simulink model "FOC_6EKF_V2"  (R2024b)
settings: Solver=ode4  StartTime=0.0  StopTime=20  FixedStep=1e-6  RelTol=1e-3
libraries: spsMosfetLib x6, simulink x4, mcbcontrolslib x4, slpidlib x3, eeGeneralControl x3, spsSeriesRLCBranchLib x2, spsPermanentMagnetSynchronousMachineLib x1, sps_lib x1, spsDCVoltageSourceLib x1
settings Model: SimulationMode=accelerator  Creator=谭恩泽  LastModifiedBy=谭恩泽

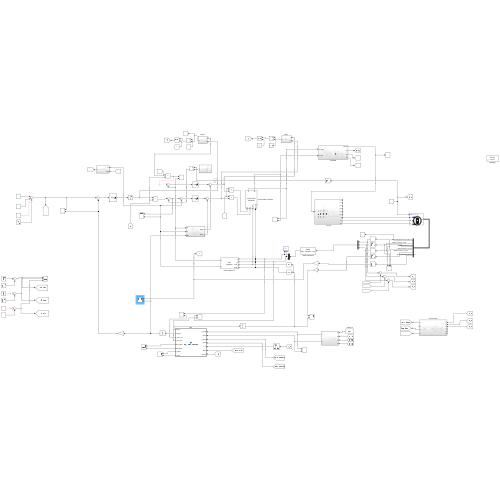
[thumbnail: Simulink's stored preview of the top-level diagram]
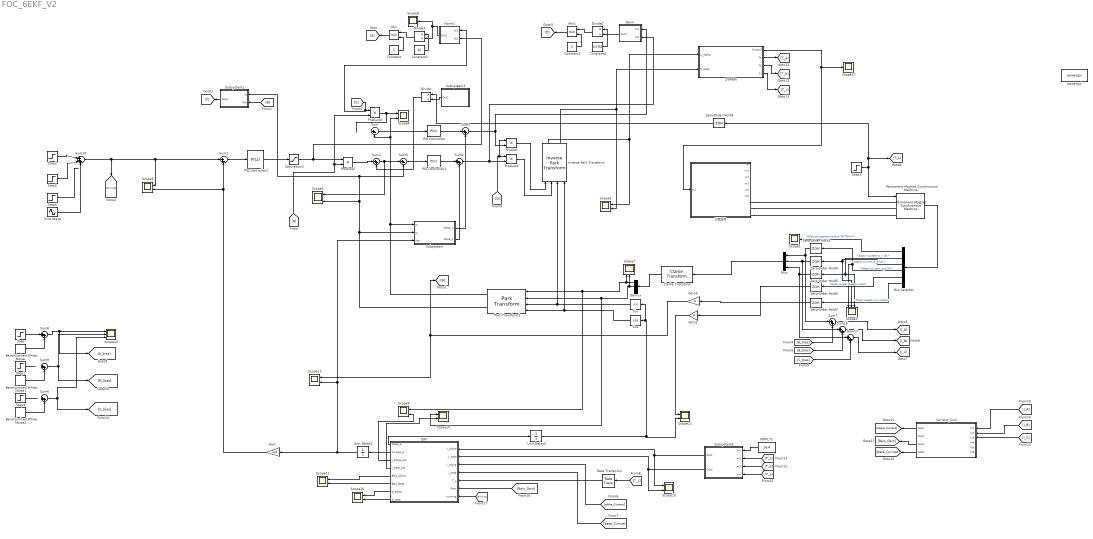
== system FOC_6EKF_V2 ==
  Band-Limited White Noise : simulink/Sources/Band-Limited White Noise  Cov=[1e-8]  Ts=1e-4  seed=[23341]
  Band-Limited White Noise1 : simulink/Sources/Band-Limited White Noise  Cov=[1e-8]  Ts=1e-4  seed=[23341]
  Band-Limited White Noise2 : simulink/Sources/Band-Limited White Noise  Cov=[1e-8]  Ts=1e-4  seed=[23341]
  Bus Selector : BusSelector  OutputSignals=Electromagnetic torque Te (N*m),Stator current is_c (A),Stator current is_b (A),Stator current is_a (A),Rotor angle thetam (rad),Rotor speed wm (rad/s)
  Clarke Transform : mcbcontrolslib/Clarke Transform  VariantControl=Variant2  PhaseInput=Three inputs  EnPowerInv=off
      settings: LibrarySourceBlock=mcblib/Controls/Math Transforms/Clarke Transform
  Constant : Constant  SampleTime=1e-4
  Constant1 : Constant  Value=20  SampleTime=1e-4
  Constant2 : Constant  SampleTime=1e-4
  Constant4 : Constant  Value=13.84  SampleTime=1e-4
  Cos : Trigonometry  Operator=cos
  Current_Sum : Subsystem
  Demux : Demux  Outputs=3
  Divide : Product  Inputs=*/  SampleTime=1e-4
  Divide1 : Product  Inputs=*/  SampleTime=1e-4
  Divide2 : Product  Inputs=*/  SampleTime=1e-4
  EKF : MATLAB Function  TreatAsAtomicUnit=on  SystemSampleTime=1e-4
  From : From
  Gain : Gain  Gain=1/4
  Gain2 : Gain  Gain=4
  Gain3 : Gain  Gain=4
  Goto : Goto
  Inverse Park Transform : mcbcontrolslib/Inverse Park Transform  PhaseInput=Two inputs  AxisAlignment=D-axis  ThetaInput=Sine and Cosine electrical position  AngleInput=Radians  N_points=1024
      settings: LibrarySourceBlock=mcblib/Controls/Math Transforms/Inverse Park Transform
  Min : MinMax  Inputs=2  SampleTime=1e-4
  Min1 : MinMax  Inputs=2  SampleTime=1e-4
  Mux : Mux  Inputs=3
  Norm : Subsystem
  Norm1 : Subsystem
  PID Controller : slpidlib/PID Controller  Controller=PI  Form=Parallel  TimeDomain=Discrete-time  UseExternalTs=off  SampleTime=1e-4  IntegratorMethod=Forward Euler  FilterMethod=Forward Euler  ControllerParametersSource=internal  P=3  I=0.5  UseKiTs=on  D=0  UseExternalDerivativeSource=off  N=100  UseFilter=on  TunerSelectOption=Transfer Function Based (PID Tuner App)  InitialConditionSource=internal  InitialConditionForIntegrator=0  InitialConditionForFilter=0  DifferentiatorICPrevScaledInput=0  ExternalReset=none  TrackingMode=off  Kt=1  LimitOutput=on  SatLimitsSource=internal  UpperSaturationLimit=15  LowerSaturationLimit=-15  LinearizeAsGain=on  AntiWindupMode=clamping  Kb=1  LimitIntegrator=off  UpperIntegratorSaturationLimit=inf  LowerIntegratorSaturationLimit=-inf  POutMin=[]  POutMax=[]  IOutMin=[]  IOutMax=[]  DOutMin=[]  DOutMax=[]  NOutMin=[]  NOutMax=[]  SumOutMin=[]  SumOutMax=[]  SaturationOutMin=[]  SaturationOutMax=[]  PParamMin=[]  PParamMax=[]  IParamMin=[]  IParamMax=[]  DParamMin=[]  DParamMax=[]  NParamMin=[]  NParamMax=[]  KbParamMin=[]  KbParamMax=[]  KtParamMin=[]  KtParamMax=[]  KbOutMin=[]  KbOutMax=[]  KtOutMin=[]  KtOutMax=[]  IntegratorOutMin=[]  IntegratorOutMax=[]  FilterOutMin=[]  FilterOutMax=[]  SumI1OutMin=[]  SumI1OutMax=[]  SumI2OutMin=[]  SumI2OutMax=[]  SumI3OutMin=[]  SumI3OutMax=[]  SumI4OutMin=[]  SumI4OutMax=[]  SumDOutMin=[]  SumDOutMax=[]  DifferentiatorOutMin=[]  DifferentiatorOutMax=[]  FilterDiffOutCoefMin=[]  FilterDiffOutCoefMax=[]  ReciprocalOutMin=[]  ReciprocalOutMax=[]  SumDenOutMin=[]  SumDenOutMax=[]  SumNumOutMin=[]  SumNumOutMax=[]  DivideOutMin=[]  DivideOutMax=[]  UdiffTsProdOutMin=[]  UdiffTsProdOutMax=[]  NTsProdOutMin=[]  NTsProdOutMax=[]  UintegralTsProdOutMin=[]  UintegralTsProdOutMax=[]  UngainTsProdOutMin=[]  UngainTsProdOutMax=[]  ClampingZeroOutDataTypeStr=Inherit: Inherit via back propagation  ClampingZeroOutMin=[]  ClampingZeroOutMax=[]  FilterDenConstantOutDataTypeStr=Inherit: Inherit via back propagation  FilterDenConstantOutMin=[]  FilterDenConstantOutMax=[]  PCopyOutDataTypeStr=Inherit: Inherit via back propagation  PCopyOutMin=[]  PCopyOutMax=[]  NCopyOutDataTypeStr=Inherit: Inherit via back propagation  NCopyOutMin=[]  NCopyOutMax=[]  IntegratorContinuousStateAttributes=''  IntegratorStateMustResolveToSignalObject=off  IntegratorRTWStateStorageClass=Auto  FilterContinuousStateAttributes=''  FilterStateMustResolveToSignalObject=off  FilterRTWStateStorageClass=Auto  ParallelPVariant=InternalParameters  IdealPVariant=Disabled  IVariant=InternalParameters  DVariant=Disabled  IntegratorVariant=Discrete  SatVariant=Enabled  AWVariant=DiscClampingParallel  PCopyVariant=Disabled  TRVariant=Disabled  FdbkBlocksVariant=Forward  IdealPFdbkVariant=Disabled  SatFdbkVariant=Disabled  DerivativeFilterVariant=Disabled  NVariant=Disabled  NCopyVariant=Disabled_SignalSpec  FilterICVariant=Disabled  IntegratorICVariant=InternalICs  ExternalResetVariant=Disabled  TRSumVariant=Passthrough  SumFdbkVariant=Disabled  SumVariant=Sum_PI  TsampFilterVariant=InternalTs  TsampNgainVariant=Passthrough  TsampIntegralVariant=Disabled_SignalSpec  ExternalSaturationOutDataTypeStr=Inherit: Same as second input  DerivativeSourceVariant=Disabled  PreIntVariant=InternalPreInt
  PID Controller1 : slpidlib/PID Controller  Controller=PI  Form=Parallel  TimeDomain=Discrete-time  UseExternalTs=off  SampleTime=1e-4  IntegratorMethod=Forward Euler  FilterMethod=Forward Euler  ControllerParametersSource=internal  P=3  I=0.5  UseKiTs=on  D=0  UseExternalDerivativeSource=off  N=100  UseFilter=on  TunerSelectOption=Transfer Function Based (PID Tuner App)  InitialConditionSource=internal  InitialConditionForIntegrator=0  InitialConditionForFilter=0  DifferentiatorICPrevScaledInput=0  ExternalReset=none  TrackingMode=off  Kt=1  LimitOutput=on  SatLimitsSource=internal  UpperSaturationLimit=15  LowerSaturationLimit=-15  LinearizeAsGain=on  AntiWindupMode=clamping  Kb=1  LimitIntegrator=off  UpperIntegratorSaturationLimit=inf  LowerIntegratorSaturationLimit=-inf  POutMin=[]  POutMax=[]  IOutMin=[]  IOutMax=[]  DOutMin=[]  DOutMax=[]  NOutMin=[]  NOutMax=[]  SumOutMin=[]  SumOutMax=[]  SaturationOutMin=[]  SaturationOutMax=[]  PParamMin=[]  PParamMax=[]  IParamMin=[]  IParamMax=[]  DParamMin=[]  DParamMax=[]  NParamMin=[]  NParamMax=[]  KbParamMin=[]  KbParamMax=[]  KtParamMin=[]  KtParamMax=[]  KbOutMin=[]  KbOutMax=[]  KtOutMin=[]  KtOutMax=[]  IntegratorOutMin=[]  IntegratorOutMax=[]  FilterOutMin=[]  FilterOutMax=[]  SumI1OutMin=[]  SumI1OutMax=[]  SumI2OutMin=[]  SumI2OutMax=[]  SumI3OutMin=[]  SumI3OutMax=[]  SumI4OutMin=[]  SumI4OutMax=[]  SumDOutMin=[]  SumDOutMax=[]  DifferentiatorOutMin=[]  DifferentiatorOutMax=[]  FilterDiffOutCoefMin=[]  FilterDiffOutCoefMax=[]  ReciprocalOutMin=[]  ReciprocalOutMax=[]  SumDenOutMin=[]  SumDenOutMax=[]  SumNumOutMin=[]  SumNumOutMax=[]  DivideOutMin=[]  DivideOutMax=[]  UdiffTsProdOutMin=[]  UdiffTsProdOutMax=[]  NTsProdOutMin=[]  NTsProdOutMax=[]  UintegralTsProdOutMin=[]  UintegralTsProdOutMax=[]  UngainTsProdOutMin=[]  UngainTsProdOutMax=[]  ClampingZeroOutDataTypeStr=Inherit: Inherit via back propagation  ClampingZeroOutMin=[]  ClampingZeroOutMax=[]  FilterDenConstantOutDataTypeStr=Inherit: Inherit via back propagation  FilterDenConstantOutMin=[]  FilterDenConstantOutMax=[]  PCopyOutDataTypeStr=Inherit: Inherit via back propagation  PCopyOutMin=[]  PCopyOutMax=[]  NCopyOutDataTypeStr=Inherit: Inherit via back propagation  NCopyOutMin=[]  NCopyOutMax=[]  IntegratorContinuousStateAttributes=''  IntegratorStateMustResolveToSignalObject=off  IntegratorRTWStateStorageClass=Auto  FilterContinuousStateAttributes=''  FilterStateMustResolveToSignalObject=off  FilterRTWStateStorageClass=Auto  ParallelPVariant=InternalParameters  IdealPVariant=Disabled  IVariant=InternalParameters  DVariant=Disabled  IntegratorVariant=Discrete  SatVariant=Enabled  AWVariant=DiscClampingParallel  PCopyVariant=Disabled  TRVariant=Disabled  FdbkBlocksVariant=Forward  IdealPFdbkVariant=Disabled  SatFdbkVariant=Disabled  DerivativeFilterVariant=Disabled  NVariant=Disabled  NCopyVariant=Disabled_SignalSpec  FilterICVariant=Disabled  IntegratorICVariant=InternalICs  ExternalResetVariant=Disabled  TRSumVariant=Passthrough  SumFdbkVariant=Disabled  SumVariant=Sum_PI  TsampFilterVariant=InternalTs  TsampNgainVariant=Passthrough  TsampIntegralVariant=Disabled_SignalSpec  ExternalSaturationOutDataTypeStr=Inherit: Same as second input  DerivativeSourceVariant=Disabled  PreIntVariant=InternalPreInt
  PID Controller2 : slpidlib/PID Controller  Controller=PI  Form=Parallel  TimeDomain=Discrete-time  UseExternalTs=off  SampleTime=1e-4  IntegratorMethod=Forward Euler  FilterMethod=Forward Euler  ControllerParametersSource=internal  P=1.2  I=0.002  UseKiTs=on  D=0  UseExternalDerivativeSource=off  N=100  UseFilter=off  TunerSelectOption=Transfer Function Based (PID Tuner App)  InitialConditionSource=internal  InitialConditionForIntegrator=0  InitialConditionForFilter=0  DifferentiatorICPrevScaledInput=0  ExternalReset=none  TrackingMode=off  Kt=1  LimitOutput=on  SatLimitsSource=internal  UpperSaturationLimit=20  LowerSaturationLimit=-20  LinearizeAsGain=on  AntiWindupMode=clamping  Kb=1  LimitIntegrator=off  UpperIntegratorSaturationLimit=inf  LowerIntegratorSaturationLimit=-inf  POutMin=[]  POutMax=[]  IOutMin=[]  IOutMax=[]  DOutMin=[]  DOutMax=[]  NOutMin=[]  NOutMax=[]  SumOutMin=[]  SumOutMax=[]  SaturationOutMin=[]  SaturationOutMax=[]  PParamMin=[]  PParamMax=[]  IParamMin=[]  IParamMax=[]  DParamMin=[]  DParamMax=[]  NParamMin=[]  NParamMax=[]  KbParamMin=[]  KbParamMax=[]  KtParamMin=[]  KtParamMax=[]  KbOutMin=[]  KbOutMax=[]  KtOutMin=[]  KtOutMax=[]  IntegratorOutMin=[]  IntegratorOutMax=[]  FilterOutMin=[]  FilterOutMax=[]  SumI1OutMin=[]  SumI1OutMax=[]  SumI2OutMin=[]  SumI2OutMax=[]  SumI3OutMin=[]  SumI3OutMax=[]  SumI4OutMin=[]  SumI4OutMax=[]  SumDOutMin=[]  SumDOutMax=[]  DifferentiatorOutMin=[]  DifferentiatorOutMax=[]  FilterDiffOutCoefMin=[]  FilterDiffOutCoefMax=[]  ReciprocalOutMin=[]  ReciprocalOutMax=[]  SumDenOutMin=[]  SumDenOutMax=[]  SumNumOutMin=[]  SumNumOutMax=[]  DivideOutMin=[]  DivideOutMax=[]  UdiffTsProdOutMin=[]  UdiffTsProdOutMax=[]  NTsProdOutMin=[]  NTsProdOutMax=[]  UintegralTsProdOutMin=[]  UintegralTsProdOutMax=[]  UngainTsProdOutMin=[]  UngainTsProdOutMax=[]  ClampingZeroOutDataTypeStr=Inherit: Inherit via back propagation  ClampingZeroOutMin=[]  ClampingZeroOutMax=[]  FilterDenConstantOutDataTypeStr=Inherit: Inherit via back propagation  FilterDenConstantOutMin=[]  FilterDenConstantOutMax=[]  PCopyOutDataTypeStr=Inherit: Inherit via back propagation  PCopyOutMin=[]  PCopyOutMax=[]  NCopyOutDataTypeStr=Inherit: Inherit via back propagation  NCopyOutMin=[]  NCopyOutMax=[]  IntegratorContinuousStateAttributes=''  IntegratorStateMustResolveToSignalObject=off  IntegratorRTWStateStorageClass=Auto  FilterContinuousStateAttributes=''  FilterStateMustResolveToSignalObject=off  FilterRTWStateStorageClass=Auto  ParallelPVariant=InternalParameters  IdealPVariant=Disabled  IVariant=InternalParameters  DVariant=Disabled  IntegratorVariant=Discrete  SatVariant=Enabled  AWVariant=DiscClampingParallel  PCopyVariant=Disabled  TRVariant=Disabled  FdbkBlocksVariant=Forward  IdealPFdbkVariant=Disabled  SatFdbkVariant=Disabled  DerivativeFilterVariant=Disabled  NVariant=Disabled  NCopyVariant=Disabled_SignalSpec  FilterICVariant=Disabled  IntegratorICVariant=InternalICs  ExternalResetVariant=Disabled  TRSumVariant=Passthrough  SumFdbkVariant=Disabled  SumVariant=Sum_PI  TsampFilterVariant=InternalTs  TsampNgainVariant=Passthrough  TsampIntegralVariant=Disabled_SignalSpec  ExternalSaturationOutDataTypeStr=Inherit: Same as second input  DerivativeSourceVariant=Disabled  PreIntVariant=InternalPreInt
  PWM_Ts : Constant  Value=1e-4  SampleTime=1e-4
  Park Transform1 : mcbcontrolslib/Park Transform  PhaseInput=Two inputs  AxisAlignment=D-axis  ThetaInput=Sine and Cosine electrical position  AngleInput=Per-unit  N_points=1024
      settings: LibrarySourceBlock=mcblib/Controls/Math Transforms/Park Transform
  Permanent Magnet Synchronous Machine : spsPermanentMagnetSynchronousMachineLib/Permanent Magnet Synchronous Machine  NbPhases=3  FluxDistribution=Sinusoidal  RotorType=Round  MechanicalLoad=Torque Tm  PresetModel=No  ShowDetailedParameters=on  MeasurementBus=off  Resistance=0.4578  Inductance=8.5e-3  dqInductances=[8.5e-3,8.5e-3]  La=0.005  MachineConstant=Flux linkage established by magnets (V.s)  Flux=0.02  VoltageCst=14.5104  TorqueCst=0.12  Flat=120  Mechanical=[0.0005 0.0003035 4 0]  PolePairs=4  InitialConditions=[0,0, 0,0]  InitialConditions5ph=[0 0 0 0 0 0]  RefAngle=Aligned with phase A axis (original Park)  IterativeDiscreteModel=Trapezoidal non iterative  TsBlock=-1  TsPowergui=0
  Product{,2..4} (4 alike) : Product  SampleTime=1e-4
  Rate Transition : RateTransition  Integrity=off  OutPortSampleTime=1e-4
  SVPWM : Subsystem
  Saturation2 : Saturate  UpperLimit=20  LowerLimit=-20
  Scope1 : Scope
  Scope{2,4..6,9..13,15..16} (11 alike) : Scope  NumInputPorts=2
  Scope14 : Scope  NumInputPorts=3
  Scope17 : Scope
  Scope3 : Scope  NumInputPorts=3
  Scope7 : Scope  NumInputPorts=3
  Scope8 : Scope
  Sin : Trigonometry
  Sine Wave : Sin  Amplitude=30  Frequency=pi  SampleTime=1e-4
  Step : Step  Time=5  SampleTime=1e-4
  Step1 : Step  Time=3  SampleTime=1e-4
  Step2 : Step  After=50  SampleTime=1e-4
  Step3 : Step  Time=0.1  After=0.001  SampleTime=1e-6
  Step4 : Step  Time=3  After=0.5  SampleTime=1e-4
  Step5 : Step  Time=2.5  After=20  SampleTime=1e-4
  Step6 : Step  Time=4  After=-40  SampleTime=1e-4
  Subsystem : Subsystem
  Subsystem1 : Subsystem
  Subsystem2 : Subsystem
  Subsystem3 : Subsystem
  Sum : Sum  Inputs=|+-  SampleTime=1e-4
  Sum1 : Sum  Inputs=|++  SampleTime=1e-4
  Sum10 : Sum  Inputs=|+++
  Sum{6..9,16..17} (6 alike) : Sum  Inputs=|++
  Sum2 : Sum  Inputs=|+-
  Sum3 : Sum  Inputs=|++  SampleTime=1e-4
  Sum4 : Sum  Inputs=|++  SampleTime=1e-4
  Sum5 : Sum  Inputs=|+-  SampleTime=1e-4
  Unit Delay1 : UnitDelay  SampleTime=-1  HasFrameUpgradeWarning=on
  Unit Delay3 : UnitDelay  SampleTime=-1  HasFrameUpgradeWarning=on
  Zero-Order Hold{3..8} (6 alike) : ZeroOrderHold  SampleTime=1e-4
  powergui : sps_lib/powergui  Priority=1  SimulationMode=Discrete  SampleTime=1e-6  frequency=60  Iterations=50  frequencyindice=0  Pbase=100e6  ErrMax=1e-4  UnitsV=kV  UnitsW=MW  buscounter=0  FunctionMessages=off  echomessages=off  EnableUseOfTLC=off  CurrentSourceSwitches=off  DisableSnubberDevices=off  DisableRonSwitches=off  DisableVfSwitches=off  DisplayEquations=off  AutomaticDiscreteSolvers=off  SolverType=Tustin/Backward Euler (TBE)  Interpol=off  ExternalGateDelay=off  methode=off  Ts=100  x0status=blocks  SPID=on  SwTol=0  HookPort=off  NonlinearTolerance=1e-4  nMaxIteration=100  ContinueOnMaxIteration=off  RestoreLinks=warning  ResistiveCurrentMeasurement=off  Frange=[0:2:500]  Ylog=off  Xlog=on  ShowGrid=off  save=off  variable=ZData  structure=0  ZoomFFT=off  StartTime=0.0  cycles=1  DisplayStyle=1  fundamental=60  FreqAxis=off  MaxFrequency=1000  frequencyindicesteady=1  RmsSteady=1  display=off
  三相逆变 : Subsystem
  wires:
  Clarke Transform/1 -> Demux/1
  Demux/2 -> Scope7/2, Park Transform1/2, Scope10/1
  Permanent Magnet Synchronous Machine/1 -> Bus Selector/1
  Bus Selector/1 -> Scope1/1  "<Electromagnetic torque Te (N*m)>"
  Bus Selector/2 -> Zero-Order Hold5/1, Scope3/3  "<Stator current is_c (A)>"
  Bus Selector/3 -> Scope3/2, Zero-Order Hold4/1  "<Stator current is_b (A)>"
  Bus Selector/4 -> Zero-Order Hold3/1, Scope3/1  "<Stator current is_a (A)>"
  Park Transform1/1 -> Subsystem/1(Id), Sum/2, Scope4/2
  Park Transform1/2 -> Scope2/2, Subsystem1/1(Iq), Sum5/2, Subsystem/2(Iq)
  Demux/1 -> Park Transform1/1, Scope9/1, Scope7/1
  Sum2/1 -> PID Controller2/1
  Sum10/1 -> Sum2/1, Scope5/1, [Running]
  Bus Selector/5 -> Zero-Order Hold6/1  "<Rotor angle thetam (rad)>"
  Gain2/1 -> Scope11/1
  Subsystem/1(dleta_d) -> Sum3/2
  PID Controller/1 -> Sum3/1
  Subsystem/2(dleta_q) -> Sum4/2
  PID Controller1/1 -> Sum4/1
  Zero-Order Hold7/1 -> Gain3/1
  Gain3/1 -> [B], Scope13/1
  Saturation2/1 -> Norm1/2(In2), Product2/1
  Step3/1 -> Zero-Order Hold8/1, [T_L], Permanent Magnet Synchronous Machine/1
  PID Controller2/1 -> Saturation2/1
  Sum4/1 -> Norm/2(In2), Product4/2
  Sum3/1 -> Norm/1(In1), Product/2
  Divide/1 -> Sum1/2
  Norm1/1(Out1) -> Divide1/2, Scope8/1
  Constant1/1 -> Divide1/1
  From/1 -> Product3/2, Product2/2
  [C] -> Product3/1, Norm1/1(In1)
  Subsystem1/1(Out1) -> [C]
  Sum/1 -> PID Controller/1
  Sum1/1 -> Scope2/1, Sum5/1
  Product2/1 -> Sum1/1
  [B] -> Subsystem1/2(We)
  Norm/1(Out1) -> Divide2/2
  Constant4/1 -> Divide2/1
  [D] -> Product/1, Product4/1
  Product/1 -> Inverse Park Transform/1
  Product4/1 -> Inverse Park Transform/2
  Divide2/1 -> Min1/1
  Divide1/1 -> Min/1
  Product3/1 -> Scope4/1
  Min/1 -> Goto/1
  Min1/1 -> [D]
  Constant/1 -> Min/2
  Constant2/1 -> Min1/2
  Sum5/1 -> PID Controller1/1
  [alpha_Current] -> EKF/3(i_alpha)
  [beta_Currnet] -> EKF/4(i_beta)
  EKF/3(i_alpha_est) -> Scope9/2
  EKF/2(omega_e) -> Unit Delay1/1
  EKF/4(i_beta_est) -> Scope10/2
  Unit Delay3/1 -> Scope11/2, Cos/1, Sin/1
  EKF/5(Bais_Alpha) -> Scope12/1
  Band-Limited White Noise/1 -> Sum8/2
  Sum8/1 -> Scope14/1, [A_bias]
  Sum9/1 -> Scope14/2, [B_bias]
  Band-Limited White Noise1/1 -> Sum9/2
  Step/1 -> Sum8/1
  Step1/1 -> ?
  [T_L] -> Rate Transition/1
  Rate Transition/1 -> EKF/5(T_L)
  Zero-Order Hold3/1 -> Sum7/1, Mux/1
  Zero-Order Hold4/1 -> Sum16/1, Mux/2
  Zero-Order Hold5/1 -> Mux/3, Sum17/1
  Mux/1 -> Clarke Transform/1
  Bus Selector/6 -> Zero-Order Hold7/1  "<Rotor speed wm (rad/s)>"
  Zero-Order Hold6/1 -> Gain2/1
  Cos/1 -> Park Transform1/4, Inverse Park Transform/4
  Sin/1 -> Park Transform1/3, Inverse Park Transform/3
  Inverse Park Transform/1 -> Scope6/1, SVPWM/1(U_alpha)
  Inverse Park Transform/2 -> SVPWM/2(U_beta), Scope6/2
  Zero-Order Hold8/1 -> Divide/1
  SVPWM/1(Control) -> 三相逆变/1(In1), Scope17/1
  SVPWM/2(Ta) -> [T_a]
  SVPWM/3(Tb) -> [T_b]
  SVPWM/4(Tc) -> [T_c]
  Step4/1 -> ?
  Sum6/1 -> Scope14/3, [C_bias]
  Band-Limited White Noise2/1 -> Sum6/2
  [A_bias] -> Sum7/2
  [B_bias] -> Sum16/2
  Sum16/1 -> [I_B]
  [C_bias] -> Sum17/2
  Sum7/1 -> [I_A]
  Sum17/1 -> [I_C]
  [Bais_Gain] -> EKF/6(Gain)
  EKF/6(Bais_Beta) -> Scope12/2
  [I_A] -> Current_Sum/1(In1)
  [I_B] -> Current_Sum/2(In2)
  [I_C] -> Current_Sum/3(In3)
  Current_Sum/1(Out1) -> [alpha_Current]
  Current_Sum/3(Out3) -> [Bais_Gain]
  Current_Sum/4(Out4) -> [beta_Currnet]
  Subsystem3/1(Out1) -> Divide/2
  EKF/1(theta_e) -> Unit Delay3/1
  PWM_Ts/1 -> Subsystem2/1(In1)
  [T_c] -> Subsystem2/2(In2)
  [T_b] -> Subsystem2/3(In3)
  Subsystem2/2(Out2) -> Scope15/2, EKF/2(v_beta)
  Subsystem2/1(Out1) -> Scope15/1, EKF/1(v_alpha)
  [T_a] -> Subsystem2/4(In4)
  EKF/7(e_alpha) -> Scope16/1
  EKF/8(e_beta) -> Scope16/2
  Gain/1 -> Sum2/2, Scope5/2
  [Running] -> EKF/7(running)
  Step2/1 -> Sum10/1
  Step5/1 -> Sum10/2
  Step6/1 -> ?
  Unit Delay1/1 -> Subsystem/3(We), Scope13/2, Gain/1
  Sine Wave/1 -> Sum10/3
  connections:
  三相逆变/RConn1 -- Permanent Magnet Synchronous Machine/LConn1
  三相逆变/RConn2 -- Permanent Magnet Synchronous Machine/LConn2
  三相逆变/RConn3 -- Permanent Magnet Synchronous Machine/LConn3

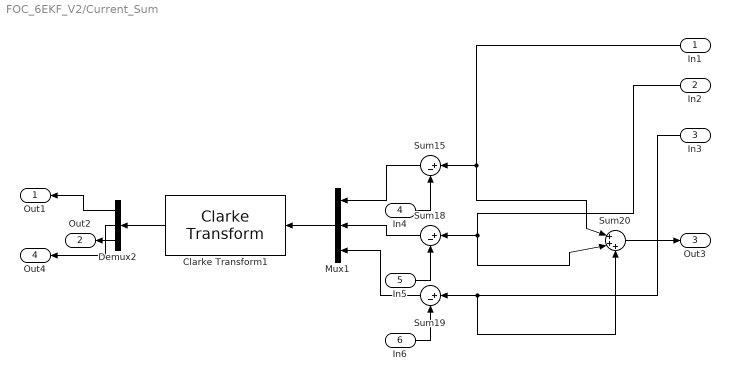
== system FOC_6EKF_V2/Current_Sum ==
  In1 : Inport
  In2 : Inport  Port=2
  In3 : Inport  Port=3
  In4 : Inport  Port=4
  In5 : Inport  Port=5
  In6 : Inport  Port=6
  Clarke Transform1 : mcbcontrolslib/Clarke Transform  VariantControl=Variant2  PhaseInput=Three inputs  EnPowerInv=off
      settings: LibrarySourceBlock=mcblib/Controls/Math Transforms/Clarke Transform
  Demux2 : Demux  Outputs=3
  Mux1 : Mux  Inputs=3
  Sum15 : Sum  Inputs=|+-
  Sum18 : Sum  Inputs=|+-
  Sum19 : Sum  Inputs=|+-
  Sum20 : Sum  Inputs=|+++
  Out1 : Outport
  Out2 : Outport  Port=2
  Out3 : Outport  Port=3
  Out4 : Outport  Port=4
  wires:
  In3/1 -> Sum20/3, Sum19/1
  Clarke Transform1/1 -> Demux2/1
  Demux2/2 -> Out4/1
  In1/1 -> Sum20/1, Sum15/1
  Mux1/1 -> Clarke Transform1/1
  Sum18/1 -> Mux1/2
  Sum19/1 -> Mux1/3
  Sum15/1 -> Mux1/1
  In2/1 -> Sum20/2, Sum18/1
  Sum20/1 -> Out3/1
  Demux2/1 -> Out1/1
  In4/1 -> Sum15/2
  In6/1 -> Sum19/2
  In5/1 -> Sum18/2
  Demux2/3 -> Out2/1

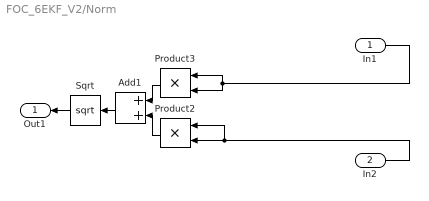
== system FOC_6EKF_V2/Norm ==
  In1 : Inport
  In2 : Inport  Port=2
  Add1 : Sum  SampleTime=1e-4
  Product2 : Product  SampleTime=1e-4
  Product3 : Product  SampleTime=1e-4
  Sqrt : Sqrt  SampleTime=1e-4
  Out1 : Outport
  wires:
  In1/1 -> Product3/1, Product3/2
  Product2/1 -> Add1/2
  In2/1 -> Product2/1, Product2/2
  Product3/1 -> Add1/1
  Add1/1 -> Sqrt/1
  Sqrt/1 -> Out1/1

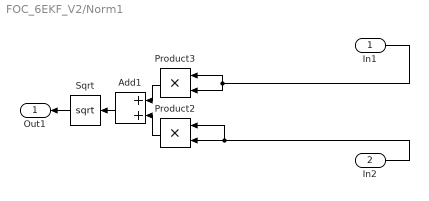
== system FOC_6EKF_V2/Norm1 ==
  In1 : Inport
  In2 : Inport  Port=2
  Add1 : Sum  SampleTime=1e-4
  Product2 : Product  SampleTime=1e-4
  Product3 : Product  SampleTime=1e-4
  Sqrt : Sqrt  SampleTime=1e-4
  Out1 : Outport
  wires:
  In1/1 -> Product3/1, Product3/2
  Product2/1 -> Add1/2
  In2/1 -> Product2/1, Product2/2
  Product3/1 -> Add1/1
  Add1/1 -> Sqrt/1
  Sqrt/1 -> Out1/1

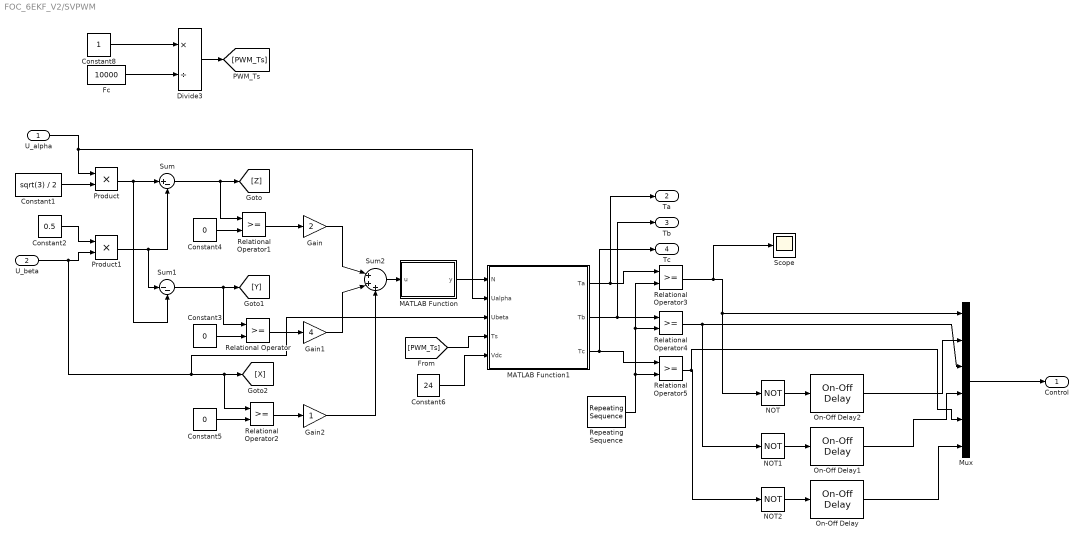
== system FOC_6EKF_V2/SVPWM ==
  U_alpha : Inport
  U_beta : Inport  Port=2
  Constant1 : Constant  Value=sqrt(3) / 2  SampleTime=1e-4
  Constant2 : Constant  Value=0.5  SampleTime=1e-4
  Constant3 : Constant  Value=0  SampleTime=1e-4
  Constant4 : Constant  Value=0  SampleTime=1e-4
  Constant5 : Constant  Value=0  SampleTime=1e-4
  Constant6 : Constant  Value=24  SampleTime=1e-4
  Constant8 : Constant  SampleTime=1e-4
  Divide3 : Product  Inputs=*/
  Fc : Constant  Value=10000  SampleTime=1e-4
  Gain : Gain  Gain=2
  Gain1 : Gain  Gain=4
  Gain2 : Gain
  MATLAB Function : MATLAB Function  TreatAsAtomicUnit=on
  MATLAB Function1 : MATLAB Function  TreatAsAtomicUnit=on  SystemSampleTime=1e-4
  Mux : Mux  Inputs=6
  NOT : Logic  Operator=NOT  IconShape=distinctive  AllPortsSameDT=off  OutDataTypeStr=boolean  SampleTime=1e-6
  NOT1 : Logic  Operator=NOT  IconShape=distinctive  AllPortsSameDT=off  OutDataTypeStr=boolean  SampleTime=1e-6
  NOT2 : Logic  Operator=NOT  IconShape=distinctive  AllPortsSameDT=off  OutDataTypeStr=boolean  SampleTime=1e-6
  On-Off Delay : eeGeneralControl/On-Off Delay  LabelModeActiveChoice=Discrete  Td_on=1e-6  Td_off=1e-6  IC=0  Ts=1e-6
      settings: LibrarySourceBlock=ee_sl_lib/General Control/On-Off Delay
  On-Off Delay1 : eeGeneralControl/On-Off Delay  LabelModeActiveChoice=Discrete  Td_on=1e-6  Td_off=1e-6  IC=0  Ts=1e-6
      settings: LibrarySourceBlock=ee_sl_lib/General Control/On-Off Delay
  On-Off Delay2 : eeGeneralControl/On-Off Delay  LabelModeActiveChoice=Discrete  Td_on=1e-6  Td_off=1e-6  IC=0  Ts=1e-6
      settings: LibrarySourceBlock=ee_sl_lib/General Control/On-Off Delay
  Product : Product
  Product1 : Product
  Relational Operator : RelationalOperator  OutDataTypeStr=boolean  RndMeth=Simplest  InputSameDT=off
  Relational Operator1 : RelationalOperator  OutDataTypeStr=boolean  RndMeth=Simplest  InputSameDT=off
  Relational Operator2 : RelationalOperator  OutDataTypeStr=boolean  RndMeth=Simplest  InputSameDT=off
  Relational Operator3 : RelationalOperator  OutDataTypeStr=boolean  SampleTime=1e-6  RndMeth=Simplest  InputSameDT=off
  Relational Operator4 : RelationalOperator  OutDataTypeStr=boolean  SampleTime=1e-6  RndMeth=Simplest  InputSameDT=off
  Relational Operator5 : RelationalOperator  OutDataTypeStr=boolean  SampleTime=1e-6  RndMeth=Simplest  InputSameDT=off
  Repeating Sequence : simulink/Sources/Repeating Sequence  rep_seq_t=[0 5e-5 1e-4]  rep_seq_y=[0 1e-4 0]
  Scope : Scope
  Sum : Sum  Inputs=|+-
  Sum1 : Sum  Inputs=|--
  Sum2 : Sum  Inputs=|+++
  Control : Outport
  Ta : Outport  Port=2
  Tb : Outport  Port=3
  Tc : Outport  Port=4
  wires:
  Fc/1 -> Divide3/2
  Divide3/1 -> [PWM_Ts]
  Constant8/1 -> Divide3/1
  U_alpha/1 -> MATLAB Function1/2(Ualpha), Product/1
  Constant1/1 -> Product/2
  Product/1 -> Sum1/2, Sum/1
  Constant2/1 -> Product1/1
  U_beta/1 -> MATLAB Function1/3(Ubeta), Relational Operator2/1, [X], Product1/2
  Product1/1 -> Sum1/1, Sum/2
  Sum/1 -> Relational Operator1/1, [Z]
  Sum1/1 -> Relational Operator/1, [Y]
  Constant3/1 -> Relational Operator/2
  Constant4/1 -> Relational Operator1/2
  Constant5/1 -> Relational Operator2/2
  Relational Operator1/1 -> Gain/1
  Relational Operator/1 -> Gain1/1
  Relational Operator2/1 -> Gain2/1
  Gain/1 -> Sum2/1
  Gain1/1 -> Sum2/2
  Gain2/1 -> Sum2/3
  Sum2/1 -> MATLAB Function/1(u)
  MATLAB Function/1(y) -> MATLAB Function1/1(N)
  Constant6/1 -> MATLAB Function1/5(Vdc)
  [PWM_Ts] -> MATLAB Function1/4(Ts)
  MATLAB Function1/1(Ta) -> Ta/1, Relational Operator3/1
  MATLAB Function1/2(Tb) -> Tb/1, Relational Operator4/1
  MATLAB Function1/3(Tc) -> Relational Operator5/1, Tc/1
  Repeating Sequence/1 -> Relational Operator3/2, Relational Operator4/2, Relational Operator5/2
  NOT2/1 -> On-Off Delay/1
  NOT1/1 -> On-Off Delay1/1
  NOT/1 -> On-Off Delay2/1
  Relational Operator3/1 -> Scope/1, NOT/1, Mux/1
  Relational Operator4/1 -> NOT1/1, Mux/3
  Relational Operator5/1 -> Mux/5, NOT2/1
  On-Off Delay2/1 -> Mux/2
  On-Off Delay1/1 -> Mux/4
  On-Off Delay/1 -> Mux/6
  Mux/1 -> Control/1

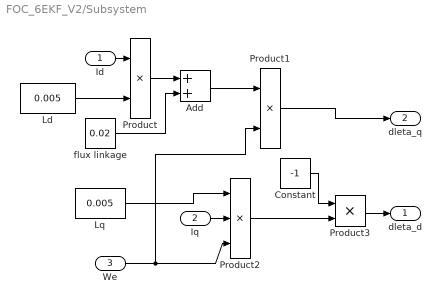
== system FOC_6EKF_V2/Subsystem ==
  Id : Inport
  Iq : Inport  Port=2
  We : Inport  Port=3
  Add : Sum  SampleTime=1e-4
  Constant : Constant  Value=-1  SampleTime=1e-4
  Ld : Constant  Value=0.005  SampleTime=1e-4
  Lq : Constant  Value=0.005  SampleTime=1e-4
  Product : Product  SampleTime=1e-4
  Product1 : Product  SampleTime=1e-4
  Product2 : Product  Inputs=3  SampleTime=1e-4
  Product3 : Product  SampleTime=1e-4
  flux linkage : Constant  Value=0.02  SampleTime=1e-4
  dleta_d : Outport
  dleta_q : Outport  Port=2
  wires:
  Iq/1 -> Product2/2
  Add/1 -> Product1/1
  Product/1 -> Add/1
  flux linkage/1 -> Add/2
  Id/1 -> Product/1
  We/1 -> Product1/2, Product2/3
  Lq/1 -> Product2/1
  Ld/1 -> Product/2
  Constant/1 -> Product3/1
  Product2/1 -> Product3/2
  Product3/1 -> dleta_d/1
  Product1/1 -> dleta_q/1

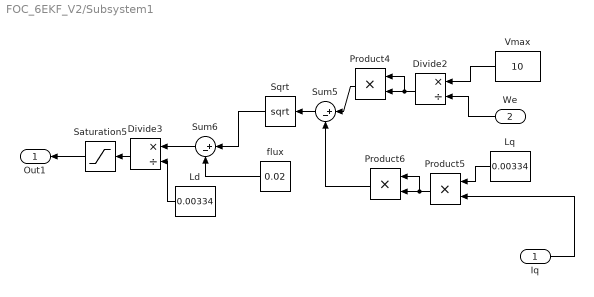
== system FOC_6EKF_V2/Subsystem1 ==
  Iq : Inport
  We : Inport  Port=2
  Divide2 : Product  Inputs=*/  SampleTime=1e-4
  Divide3 : Product  Inputs=*/  SampleTime=1e-4
  Ld : Constant  Value=0.00334  SampleTime=1e-4
  Lq : Constant  Value=0.00334  SampleTime=1e-4
  Product4 : Product  SampleTime=1e-4
  Product5 : Product  SampleTime=1e-4
  Product6 : Product  SampleTime=1e-4
  Saturation5 : Saturate  UpperLimit=0  LowerLimit=-10  SampleTime=1e-4
  Sqrt : Sqrt  OutputSignalType=real  SampleTime=1e-4
  Sum5 : Sum  Inputs=|+-  SampleTime=1e-4
  Sum6 : Sum  Inputs=|+-  SampleTime=1e-4
  Vmax : Constant  Value=10  SampleTime=1e-4
  flux : Constant  Value=0.02  SampleTime=1e-4
  Out1 : Outport
  wires:
  Sum6/1 -> Divide3/1
  Vmax/1 -> Divide2/1
  Divide2/1 -> Product4/1, Product4/2
  Product5/1 -> Product6/1, Product6/2
  Product4/1 -> Sum5/1
  We/1 -> Divide2/2
  Ld/1 -> Divide3/2
  Iq/1 -> Product5/2
  Sum5/1 -> Sqrt/1
  flux/1 -> Sum6/2
  Product6/1 -> Sum5/2
  Divide3/1 -> Saturation5/1
  Lq/1 -> Product5/1
  Sqrt/1 -> Sum6/1
  Saturation5/1 -> Out1/1

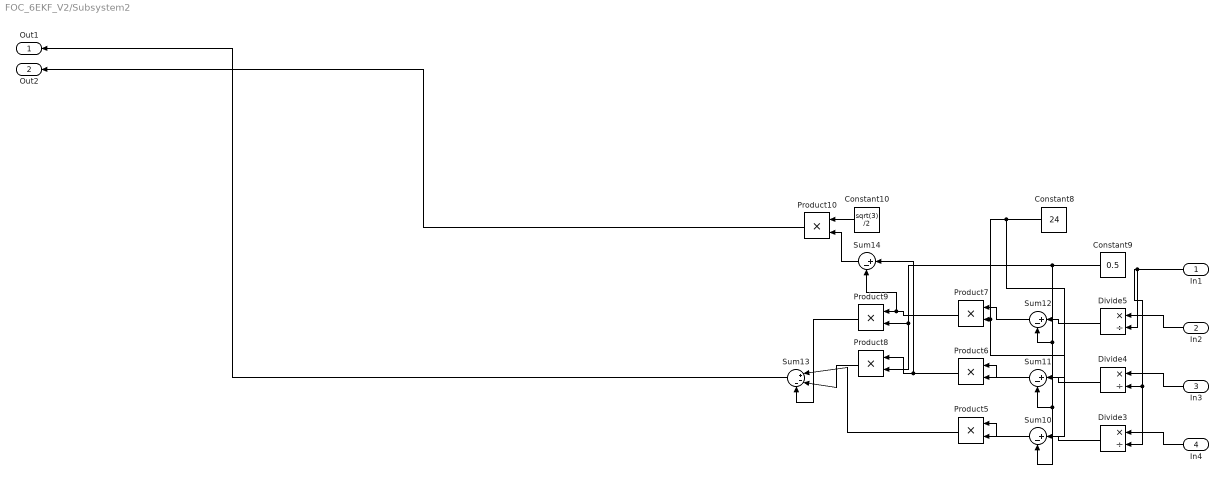
== system FOC_6EKF_V2/Subsystem2 ==
  In1 : Inport
  In2 : Inport  Port=2
  In3 : Inport  Port=3
  In4 : Inport  Port=4
  Constant10 : Constant  Value=sqrt(3) /2  SampleTime=1e-4
  Constant8 : Constant  Value=24  SampleTime=1e-4
  Constant9 : Constant  Value=0.5  SampleTime=1e-4
  Divide3 : Product  Inputs=*/
  Divide4 : Product  Inputs=*/
  Divide5 : Product  Inputs=*/
  Product{5..10} (6 alike) : Product
  Sum{10..12,14} (4 alike) : Sum  Inputs=|+-
  Sum13 : Sum  Inputs=|+--
  Out1 : Outport
  Out2 : Outport  Port=2
  wires:
  In1/1 -> Divide4/2, Divide3/2, Divide5/2
  Sum10/1 -> Product5/1
  Sum14/1 -> Product10/2
  In2/1 -> Divide5/1
  Sum12/1 -> Product7/1
  Product7/1 -> Sum14/2, Product9/1
  Divide5/1 -> Sum12/1
  Product6/1 -> Sum14/1, Product8/1
  Sum13/1 -> Out1/1
  Product5/1 -> Sum13/1
  Product8/1 -> Sum13/2
  Product9/1 -> Sum13/3
  Constant8/1 -> Product6/2, Product7/2, Product5/2
  Constant9/1 -> Sum11/2, Sum10/2, Sum12/2, Product9/2, Product8/2
  Product10/1 -> Out2/1
  Sum11/1 -> Product6/1
  Divide3/1 -> Sum10/1
  Divide4/1 -> Sum11/1
  Constant10/1 -> Product10/1
  In3/1 -> Divide4/1
  In4/1 -> Divide3/1

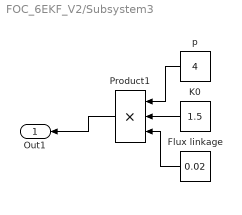
== system FOC_6EKF_V2/Subsystem3 ==
  Flux linkage : Constant  Value=0.02  SampleTime=1e-4
  K0 : Constant  Value=1.5  SampleTime=1e-4
  Product1 : Product  Inputs=3
  p : Constant  Value=4  SampleTime=1e-4
  Out1 : Outport
  wires:
  Flux linkage/1 -> Product1/3
  p/1 -> Product1/1
  K0/1 -> Product1/2
  Product1/1 -> Out1/1

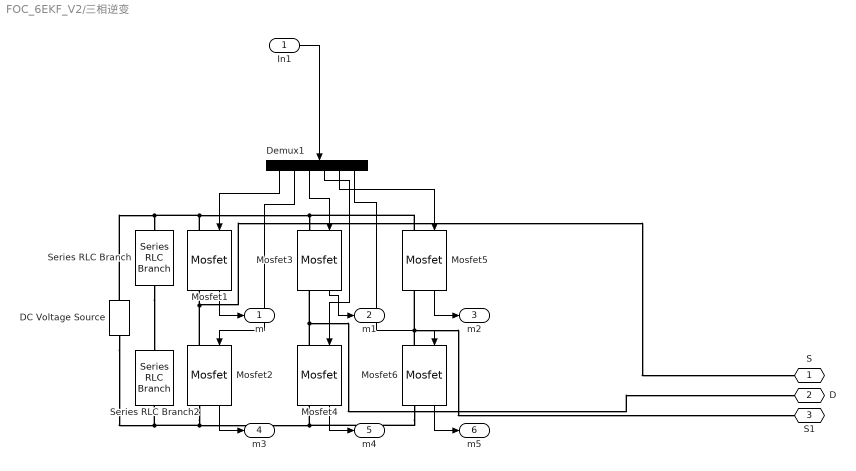
== system FOC_6EKF_V2/三相逆变 ==
  In1 : Inport
  DC Voltage Source : spsDCVoltageSourceLib/DC Voltage Source  Amplitude=24  Measurements=Voltage
  Demux1 : Demux  Outputs=6
      settings: DisplayOption=none
  Mosfet{1..6} (6 alike) : spsMosfetLib/Mosfet  Ron=0.1  Lon=0  Rd=0.01  Vfd=0.8  IC=0  Rs=50  Cs=4.7e-9  Measurements=on
  Series RLC Branch : spsSeriesRLCBranchLib/Series RLC Branch  LConnTagsString=__new0  RConnTagsString=__new0  BranchType=RC  Resistance=0.01  Inductance=1e-3  SetiL0=off  InitialCurrent=0  Capacitance=1e-3  Setx0=off  InitialVoltage=0  Measurements=None
  Series RLC Branch2 : spsSeriesRLCBranchLib/Series RLC Branch  LConnTagsString=__new0  RConnTagsString=__new0  BranchType=RC  Resistance=0.01  Inductance=1e-3  SetiL0=off  InitialCurrent=0  Capacitance=1e-3  Setx0=off  InitialVoltage=0  Measurements=None
  S : PMIOPort  Side=Right
  D : PMIOPort  Port=2  Side=Right
  S1 : PMIOPort  Port=3  Side=Right
  m : Outport
  m1 : Outport  Port=2
  m2 : Outport  Port=3
  m3 : Outport  Port=4
  m4 : Outport  Port=5
  m5 : Outport  Port=6
  wires:
  Mosfet6/1 -> m5/1
  Demux1/6 -> Mosfet6/1
  Demux1/1 -> Mosfet1/1
  Demux1/3 -> Mosfet3/1
  Mosfet1/1 -> m/1
  Mosfet2/1 -> m3/1
  Demux1/4 -> Mosfet4/1
  Demux1/2 -> Mosfet2/1
  In1/1 -> Demux1/1
  Demux1/5 -> Mosfet5/1
  Mosfet3/1 -> m1/1
  Mosfet5/1 -> m2/1
  Mosfet4/1 -> m4/1
  connections:
  Mosfet5/LConn1 -- Mosfet1/LConn1 -- DC Voltage Source/RConn1 -- Series RLC Branch/LConn1 -- Mosfet3/LConn1
  Mosfet6/LConn1 -- S1/RConn1 -- Mosfet5/RConn1
  Mosfet6/RConn1 -- Mosfet2/RConn1 -- DC Voltage Source/LConn1 -- Series RLC Branch2/RConn1 -- Mosfet4/RConn1
  Mosfet2/LConn1 -- S/RConn1 -- Mosfet1/RConn1
  Mosfet3/RConn1 -- D/RConn1 -- Mosfet4/LConn1
  Series RLC Branch/RConn1 -- Series RLC Branch2/LConn1

== matlab function FOC_6EKF_V2/SVPWM/MATLAB Function ==
  data: u input; y output
function y = tab(u)

switch u
    case 1
        y = 2;
    case 2
        y = 6;
    case 3
        y = 1;
    case 4
        y = 4;
    case 5
        y = 3;
    case 6
        y = 5;
    otherwise
        y = 0;
end

== matlab function FOC_6EKF_V2/EKF ==
  settings: updateMethod=DISCRETE
  data: v_alpha input; theta_e output; v_beta input; i_alpha input; i_beta input; omega_e output; i_alpha_est output; i_beta_est output; Bais_Alpha output; T_L input; Gain input; Bais_Beta output; e_alpha output; e_beta output; running input
function [theta_e, omega_e, i_alpha_est, i_beta_est, Bais_Alpha,Bais_Beta,e_alpha,e_beta] = ...
    ekf_pmsm_observer(v_alpha, v_beta, i_alpha, i_beta, T_L, Gain,running)
%#codegen
% 6-state EKF with sensor bias estimation
% x = [i_alpha; i_beta; omega_e; theta_e; bias_alpha; bias_beta]


persistent x_est P 

if isempty(x_est) 
    x_est = [0;0;0;0;0;0];
    P = diag([1e5, 1e5 ,1e5, 1e5, 10, 10]);
end


% ========== 电机参数 ==========
Ts = 1e-4;
Rs = 0.4578;
Ls = 0.005;
psi_f = 0.02 ;

p = 4;
J = 0.0005;
B = 0.0003035;

a = Rs / Ls;
b = psi_f / Ls;
c = 1 / Ls;
Kt = 1.5 * p * p * psi_f / J;

if running ~= 0

% ========== 噪声协方差 ==========
if Gain >0.01
Q_bais = Gain * 1e5;
else
Q_bais = 0;
end
Q = diag([1e8, 1e8, 1e1, 1e0, Q_bais, Q_bais]);

R = diag([0.01, 0.01]);

% ========== 读取状态 ==========
i_a = x_est(1); i_b = x_est(2);
w   = x_est(3); th  = x_est(4);
b_a = x_est(5); b_b = x_est(6);

sin_th = sin(th);
cos_th = cos(th);

% ========== 预测 ==========
i_a_next = i_a + Ts * (-a*i_a + b*w*sin_th + c*v_alpha);
i_b_next = i_b + Ts * (-a*i_b - b*w*cos_th + c*v_beta);

Te = 1.5 * p * psi_f * (-i_a*sin_th + i_b*cos_th);
wm = w / p;
w_next  = w + Ts * p * (Te - T_L - B*wm) / J;
th_next = th + Ts * w;
b_a_next = b_a;
b_b_next = b_b;

x_pred = [i_a_next; i_b_next; w_next; th_next; b_a_next; b_b_next];

% ========== 雅可比 (6x6) ==========
F = eye(6);

F(1,1) = 1 - Ts*a;
F(1,3) =  Ts*b*sin_th;
F(1,4) =  Ts*b*w*cos_th;

F(2,2) = 1 - Ts*a;
F(2,3) = -Ts*b*cos_th;
F(2,4) =  Ts*b*w*sin_th;

F(3,1) = -Ts*Kt*sin_th;
F(3,2) =  Ts*Kt*cos_th;
F(3,3) = 1 - Ts*B/J;
F(3,4) = -Ts*Kt*(i_a*cos_th + i_b*sin_th);

F(4,3) = Ts;

% ========== 测量更新 ==========
H = [1 0 0 0 1 0;
     0 1 0 0 0 1];

P_pred = F * P * F' + Q;

y_pred = [x_pred(1) + x_pred(5);
          x_pred(2) + x_pred(6)];

y = [i_alpha; i_beta];
residual = y - y_pred;

S = H * P_pred * H' + R;
K = P_pred * H' / S;

x_est = x_pred + K * residual;

% Joseph 协方差
I6 = eye(6);
P = (I6 - K*H) * P_pred * (I6 - K*H)' + K * R * K';
P = (P + P') / 2;

w_abs = abs(x_est(3));
if w_abs > 5.0
    emf_alpha = -sin(x_est(4));
    emf_beta  =  cos(x_est(4));
    cross_re = residual(1)*emf_beta - residual(2)*emf_alpha;
    Kp_pll = 200;
    Ki_pll = 8000;
    x_est(4) = x_est(4) + Kp_pll * Ts * cross_re;
    x_est(3) = x_est(3) + Ki_pll * Ts * cross_re;
end

end

% 防塌缩 + 限上限
P_min = [1e-14; 1e-14; 1e-14; 1e-12; 1e-8; 1e-8];
P_max = [1e14; 1e14; 1e14; 1e12; 1e8; 1e8];
for i = 1:6
    if P(i,i) < P_min(i)
        P(i,i) = P_min(i);
    end
    if P(i,i) > P_max(i)
        P(i,i) = P_max(i);
    end
end

x_est(3) = max(min(x_est(3), 3000), -3000);
x_est(4) = mod(x_est(4),2*pi);
x_est(5) = max(min(x_est(5), 1), -1);
x_est(6) = max(min(x_est(6), 1), -1);



% ========== 输出 ==========
i_alpha_est = x_est(1);
i_beta_est  = x_est(2);
omega_e     = x_est(3);
theta_e     = x_est(4);
Bais_Alpha = x_est(5);
Bais_Beta = x_est(6);
e_alpha = -x_est(3)*psi_f*sin(x_est(4));
e_beta = x_est(3)*psi_f*cos(x_est(4));
end

== matlab function FOC_6EKF_V2/SVPWM/MATLAB Function1 ==
  data: N input; Ta output; Ualpha input; Ubeta input; Ts input; Vdc input; Tb output; Tc output
function [Ta, Tb, Tc] = SVPWM_TaTbTc(N, Ualpha, Ubeta, Ts, Vdc)

sqrt3 = sqrt(3);
X = (sqrt3 * Ubeta) * Ts;
Y = ( (3/2)*Ualpha + (sqrt3/2)*Ubeta ) * Ts;
Z = ( (-3/2)*Ualpha + (sqrt3/2)*Ubeta ) * Ts;

% T1,T2 from volt-second balance
switch N
    case 1  
        T1 = -Z; T2 = X;
    case 2  
        T1 = Y; T2 = Z;
    case 3  
        T1 = X; T2 = -Y;
    case 4  
        T1 = Z; T2 = -X;
    case 5  
        T1 = -Y; T2 = -Z;
    case 6  
        T1 = -X; T2 = Y;
    otherwise
        T1 = 0; T2 = 0;
end

% Overmodulation clamp
T1 = max(T1, 0);
T2 = max(T2, 0);
Tsum = T1 + T2;
if Tsum > Ts
    T1 = T1 * Ts / Tsum;
    T2 = T2 * Ts / Tsum;
    T0 = 0;
else
    T0 = Ts - Tsum;
end


T0_half = T0 / 2;
Tcm1 = T0_half / 2;            % T0/4
Tcm2 = Tcm1 + T1 / 2;
Tcm3 = Tcm2 + T2 / 2;


switch N
    case 1  
        Ta = Ts - 2 * Tcm1;
        Tb = Ts - 2 * Tcm2;
        Tc = Ts - 2 * Tcm3;
    case 2  
        Ta = Ts - 2 * Tcm2;
        Tb = Ts - 2 * Tcm1;
        Tc = Ts - 2 * Tcm3;
    case 3  
        Ta = Ts - 2 * Tcm3;
        Tb = Ts - 2 * Tcm1;
        Tc = Ts - 2 * Tcm2;
    case 4  
        Ta = Ts - 2 * Tcm3;
        Tb = Ts - 2 * Tcm2;
        Tc = Ts - 2 * Tcm1;
    case 5  
        Ta = Ts - 2 * Tcm2;
        Tb = Ts - 2 * Tcm3;
        Tc = Ts - 2 * Tcm1;
    case 6  
        Ta = Ts - 2 * Tcm1;
        Tb = Ts - 2 * Tcm3;
        Tc = Ts - 2 * Tcm2;
    otherwise
        Ta = 0; Tb = 0; Tc = 0;
end

Ta = min(max(Ta, 0), Ts);
Tb = min(max(Tb, 0), Ts);
Tc = min(max(Tc, 0), Ts);

end
